simulink model "question3"  (R2018b)
settings: Solver=VariableStepAuto  StartTime=0.0  StopTime=0.1  RelTol=1e-3
libraries: powerlib x18
settings Model: Creator=hamza  LastModifiedBy=hamza

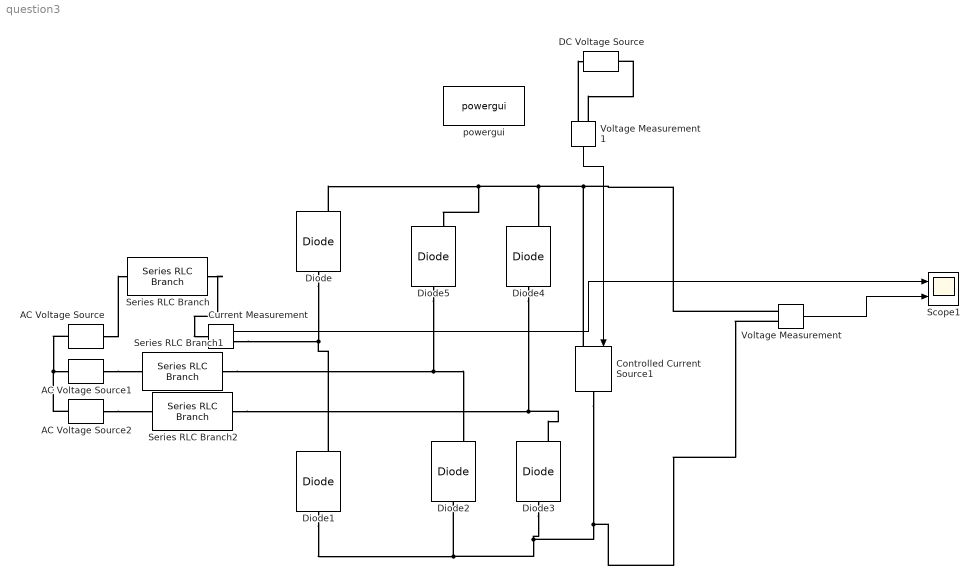
== system question3 ==
  AC Voltage Source : powerlib/Electrical Sources/AC Voltage Source  Amplitude=325.2  Phase=0  Frequency=50  SampleTime=0  Measurements=None  BusType=swing  Pref=10e3  Qref=0  Qmin=-inf  Qmax=+inf
  AC Voltage Source1 : powerlib/Electrical Sources/AC Voltage Source  Amplitude=325.2  Phase=120  Frequency=50  SampleTime=0  Measurements=None  BusType=swing  Pref=10e3  Qref=0  Qmin=-inf  Qmax=+inf
  AC Voltage Source2 : powerlib/Electrical Sources/AC Voltage Source  Amplitude=325.2  Phase=-120  Frequency=50  SampleTime=0  Measurements=None  BusType=swing  Pref=10e3  Qref=0  Qmin=-inf  Qmax=+inf
  Controlled Current Source1 : powerlib/Electrical Sources/Controlled Current Source  Initialize=on  Source_Type=DC  Amplitude=40  Phase=0  Frequency=0  Measurements=None
  Current Measurement : powerlib/Measurements/Current Measurement  PhasorSimulation=off  OutputType=Complex  PSBequivalent=0
  DC Voltage Source : powerlib/Electrical Sources/DC Voltage Source  Amplitude=40  Measurements=None
  Diode{,1..5} (6 alike) : powerlib/Power Electronics/Diode  Ron=0.001  Lon=0  Vf=0  IC=0  UseSnubber=0  Rs=500  Cs=250e-9  Measurements=on
  Scope1 : Scope  NumInputPorts=2
  Series RLC Branch : powerlib/Elements/Series RLC Branch  LConnTagsString=__new0  RConnTagsString=__new0  BranchType=L  Resistance=1  Inductance=1e-3  SetiL0=off  InitialCurrent=0  Capacitance=1e-6  Setx0=off  InitialVoltage=0  Measurements=None
  Series RLC Branch1 : powerlib/Elements/Series RLC Branch  LConnTagsString=__new0  RConnTagsString=__new0  BranchType=L  Resistance=1  Inductance=1e-3  SetiL0=off  InitialCurrent=0  Capacitance=1e-6  Setx0=off  InitialVoltage=0  Measurements=None
  Series RLC Branch2 : powerlib/Elements/Series RLC Branch  LConnTagsString=__new0  RConnTagsString=__new0  BranchType=L  Resistance=1  Inductance=1e-3  SetiL0=off  InitialCurrent=0  Capacitance=1e-6  Setx0=off  InitialVoltage=0  Measurements=None
  Voltage Measurement : powerlib/Measurements/Voltage Measurement  PhasorSimulation=off  OutputType=Complex  PSBequivalent=0
  Voltage Measurement1 : powerlib/Measurements/Voltage Measurement  PhasorSimulation=off  OutputType=Complex  PSBequivalent=0
  powergui : powerlib/powergui  Priority=1  SimulationMode=Continuous  SampleTime=50e-6  frequency=60  Iterations=50  frequencyindice=0  Pbase=100e6  ErrMax=1e-4  UnitsV=kV  UnitsW=MW  buscounter=0  FunctionMessages=off  echomessages=off  EnableUseOfTLC=off  CurrentSourceSwitches=off  DisableSnubberDevices=off  DisableRonSwitches=off  DisableVfSwitches=off  DisplayEquations=off  SolverType=Tustin/Backward Euler (TBE)  Interpol=off  ExternalGateDelay=off  methode=off  Ts=100  x0status=blocks  SPID=on  SwTol=0  HookPort=off  RestoreLinks=warning  ResistiveCurrentMeasurement=off  Frange=[0:2:500]  Ylog=off  Xlog=on  ShowGrid=off  save=off  variable=ZData  structure=0  ZoomFFT=off  StartTime=0.0  cycles=1  DisplayStyle=1  fundamental=60  FreqAxis=off  MaxFrequency=1000  frequencyindicesteady=1  RmsSteady=1  display=off
  wires:
  Voltage Measurement/1 -> Scope1/2
  Current Measurement/1 -> Scope1/1
  Voltage Measurement1/1 -> Controlled Current Source1/1
  connections:
  Current Measurement/RConn1 -- Diode1/RConn1 -- Diode/LConn1
  Voltage Measurement/LConn2 -- Controlled Current Source1/RConn1 -- Diode3/LConn1 -- Diode1/LConn1 -- Diode2/LConn1
  Voltage Measurement/LConn1 -- Controlled Current Source1/LConn1 -- Diode4/RConn1 -- Diode5/RConn1 -- Diode/RConn1
  AC Voltage Source/LConn1 -- AC Voltage Source2/LConn1 -- AC Voltage Source1/LConn1
  Voltage Measurement1/LConn1 -- DC Voltage Source/RConn1
  Voltage Measurement1/LConn2 -- DC Voltage Source/LConn1
  AC Voltage Source/RConn1 -- Series RLC Branch/LConn1
  Series RLC Branch2/RConn1 -- Diode4/LConn1 -- Diode3/RConn1
  Series RLC Branch1/RConn1 -- Diode5/LConn1 -- Diode2/RConn1
  Series RLC Branch/RConn1 -- Current Measurement/LConn1
  AC Voltage Source1/RConn1 -- Series RLC Branch1/LConn1
  AC Voltage Source2/RConn1 -- Series RLC Branch2/LConn1
